simulink model "Model_accum"  (R2024a)
settings: Solver=FixedStepAuto  StartTime=0.0  StopTime=2000  RelTol=1e-3
undefined symbols (not defined in the file or in its folder): air_density, air_din_visc, air_pr, air_pr50, air_rashod, air_transmit, d, D, i_ph, L, lambda_alum, rho, Rzagr, TAM_spec_heat, thickness, vel_crist
settings Model: Creator=User  LastModifiedBy=User

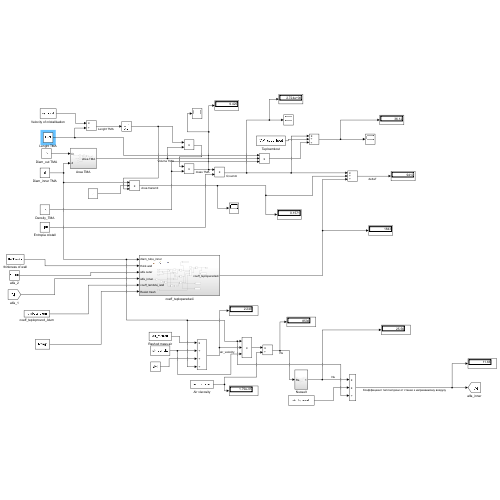
[thumbnail: Simulink's stored preview of the top-level diagram]
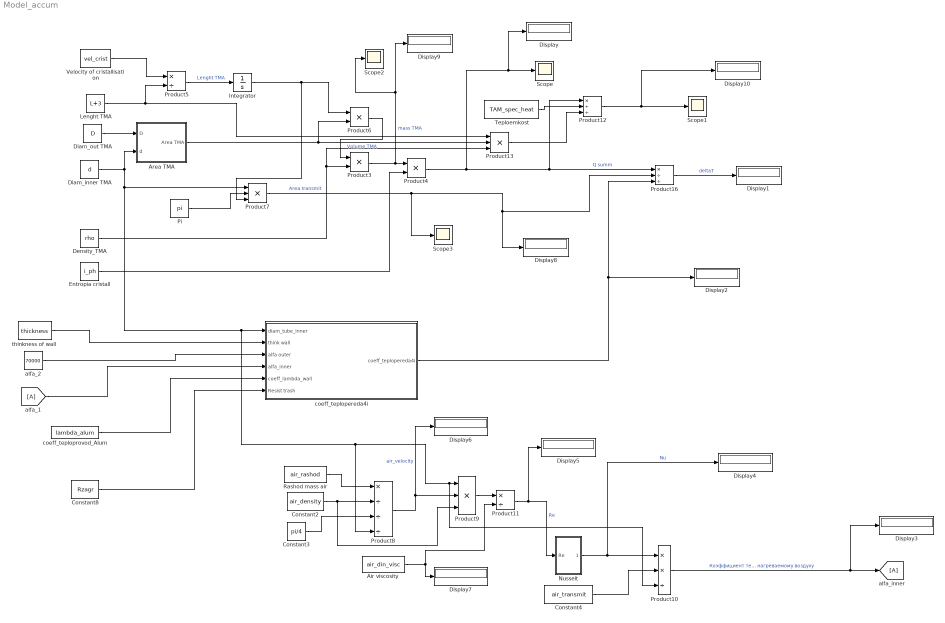
== system Model_accum ==
  Air viscosity : Constant  Value=air_din_visc
  Area TMA : Subsystem
  Constant2 : Constant  Value=air_density
  Constant3 : Constant  Value=pi/4
  Constant4 : Constant  Value=air_transmit
  Constant8 : Constant  Value=Rzagr
  Density_TMA : Constant  Value=rho
  Diam_inner TMA : Constant  Value=d
  Diam_out TMA : Constant  Value=D
  Display{,1..10} (11 alike) : Display
  Entropia cristall : Constant  Value=i_ph
  Integrator : Integrator  InitialCondition=0.001  LimitOutput=on  UpperSaturationLimit=1
  Lenght TMA : Constant  Value=L+3
  Nusselt : Subsystem
  Pi : Constant  Value=pi  OutDataTypeStr=Inherit: Inherit via back propagation
  Product10 : Product  Inputs=**/
  Product11 : Product  Inputs=*/
  Product12 : Product  Inputs=*//
  Product13 : Product  Inputs=3
  Product16 : Product  Inputs=*//
  Product3 : Product
  Product4 : Product
  Product5 : Product  Inputs=*/
  Product6 : Product
  Product7 : Product  Inputs=3
  Product8 : Product  Inputs=*///
  Product9 : Product  Inputs=3
  Rashod mass air : Constant  Value=air_rashod
  Scope{,1..3} (4 alike) : Scope
  Teploemkost : Constant  Value=TAM_spec_heat
  Velocity of cristallisation : Constant  Value=vel_crist
  alfa_1 : From
  alfa_2 : Constant  Value=70000
  alfa_inner : Goto
  coeff_teplopereda4i : Subsystem
  coeff_teploprovod_Alum : Constant  Value=lambda_alum
  thinkness of wall : Constant  Value=thickness
  wires:
  Lenght TMA/1 -> Product13/1, Product5/2
  Area TMA/1(Area TMA) -> Product6/2, Product13/2  "Volume TMA"
  Density_TMA/1 -> Product13/3, Product3/2
  Product3/1 -> Scope2/1, Display9/1, Product4/1  "mass TMA"
  Entropia cristall/1 -> Product4/2
  Product4/1 -> Product12/1, Product16/1, Scope/1, Display/1  "Q summ"
  Velocity of cristallisation/1 -> Product5/1
  Product5/1 -> Integrator/1  "Lenght TMA"
  Integrator/1 -> Product7/3, Product6/1
  Product6/1 -> Product3/1
  Product7/1 -> Scope3/1, Display8/1, Product16/2  "Area transmit"
  Product16/1 -> Display1/1  "deltaT"
  coeff_teplopereda4i/1(coeff_teplopereda4i) -> Product16/3, Display2/1
  thinkness of wall/1 -> coeff_teplopereda4i/2(think wall)
  alfa_2/1 -> coeff_teplopereda4i/3(alfa outer)
  alfa_1/1 -> coeff_teplopereda4i/4(alfa_inner)
  coeff_teploprovod_Alum/1 -> coeff_teplopereda4i/5(coeff_lambda_wall)
  Constant8/1 -> coeff_teplopereda4i/6(Resist trash)
  Diam_inner TMA/1 -> Product10/3, Product9/1, Product8/4, coeff_teplopereda4i/1(diam_tube_inner), Product7/1, Area TMA/2(d)
  Rashod mass air/1 -> Product8/1
  Constant2/1 -> Product9/3, Product8/2
  Constant3/1 -> Product8/3
  Product8/1 -> Display6/1, Product9/2  "air_velocity"
  Air viscosity/1 -> Product11/2, Display7/1
  Product11/1 -> Nusselt/1(Re), Display5/1  "Re"
  Nusselt/1(Out1) -> Display4/1, Product10/1  "Nu"
  Constant4/1 -> Product10/2
  Product10/1 -> alfa_inner/1, Display3/1  "Коэффициент теплоотдачи от стенки к нагреваемому воздуху"
  Product9/1 -> Product11/1
  Pi/1 -> Product7/2
  Teploemkost/1 -> Product12/2
  Product13/1 -> Product12/3
  Product12/1 -> Display10/1, Scope1/1
  Diam_out TMA/1 -> Area TMA/1(D)

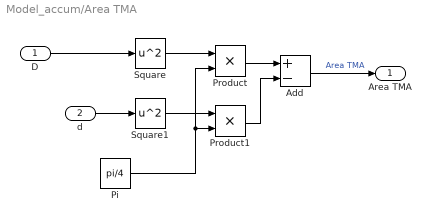
== system Model_accum/Area TMA ==
  D : Inport
  d : Inport  Port=2
  Add : Sum  Inputs=+-
  Pi : Constant  Value=pi/4  OutDataTypeStr=Inherit: Inherit via back propagation
  Product : Product
  Product1 : Product
  Square : Math  Operator=square
  Square1 : Math  Operator=square
  Area TMA : Outport
  wires:
  Square1/1 -> Product1/1
  Pi/1 -> Product/2, Product1/2
  Product1/1 -> Add/2
  D/1 -> Square/1
  Square/1 -> Product/1
  Add/1 -> Area TMA/1  "Area TMA"
  Product/1 -> Add/1
  d/1 -> Square1/1

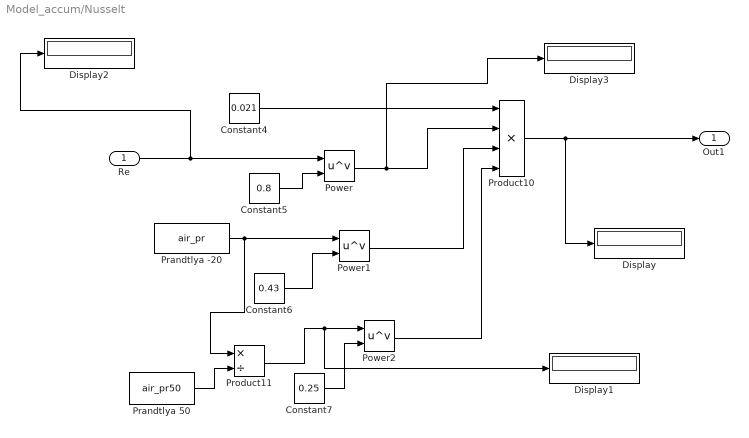
== system Model_accum/Nusselt ==
  Re : Inport
  Constant4 : Constant  Value=0.021
  Constant5 : Constant  Value=0.8
  Constant6 : Constant  Value=0.43
  Constant7 : Constant  Value=0.25
  Display{,1..3} (4 alike) : Display
  Power : Math  Operator=pow
  Power1 : Math  Operator=pow
  Power2 : Math  Operator=pow
  Prandtlya -20 : Constant  Value=air_pr
  Prandtlya 50 : Constant  Value=air_pr50
  Product10 : Product  Inputs=4
  Product11 : Product  Inputs=*/
  Out1 : Outport
  wires:
  Prandtlya -20/1 -> Product11/1, Power1/1
  Constant4/1 -> Product10/1
  Prandtlya 50/1 -> Product11/2
  Power1/1 -> Product10/3
  Constant5/1 -> Power/2
  Product11/1 -> Display1/1, Power2/1
  Power/1 -> Display3/1, Product10/2
  Constant6/1 -> Power1/2
  Constant7/1 -> Power2/2
  Power2/1 -> Product10/4
  Product10/1 -> Display/1, Out1/1
  Re/1 -> Display2/1, Power/1

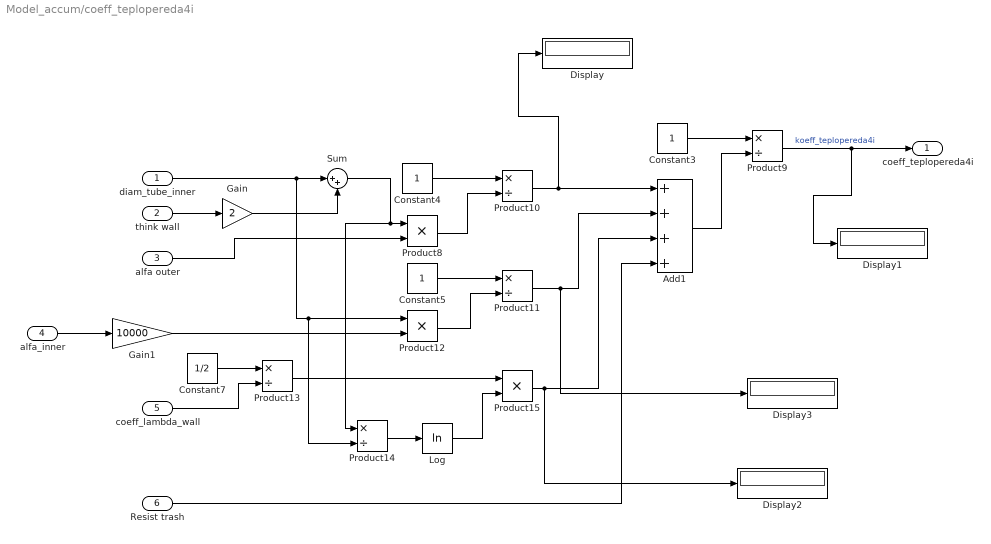
== system Model_accum/coeff_teplopereda4i ==
  diam_tube_inner : Inport
  think wall : Inport  Port=2
  alfa outer : Inport  Port=3
  alfa_inner : Inport  Port=4
  coeff_lambda_wall : Inport  Port=5
  Resist trash : Inport  Port=6
  Add1 : Sum  Inputs=++++
  Constant3 : Constant
  Constant4 : Constant
  Constant5 : Constant
  Constant7 : Constant  Value=1/2
  Display{,1..3} (4 alike) : Display
  Gain : Gain  Gain=2
  Gain1 : Gain  Gain=10000
  Log : Math  Operator=log
  Product{9..11,13..14} (5 alike) : Product  Inputs=*/
  Product12 : Product
  Product15 : Product
  Product8 : Product
  Sum : Sum  Inputs=|++
  coeff_teplopereda4i : Outport
  wires:
  diam_tube_inner/1 -> Product14/2, Product12/1, Sum/1
  Constant3/1 -> Product9/1
  think wall/1 -> Gain/1
  alfa_inner/1 -> Gain1/1
  Log/1 -> Product15/2
  Product13/1 -> Product15/1
  Product11/1 -> Display3/1, Add1/2
  Sum/1 -> Product14/1, Product8/1
  Resist trash/1 -> Add1/4
  Constant4/1 -> Product10/1
  Product12/1 -> Product11/2
  coeff_lambda_wall/1 -> Product13/2
  Product8/1 -> Product10/2
  Constant7/1 -> Product13/1
  Constant5/1 -> Product11/1
  Add1/1 -> Product9/2
  Product15/1 -> Display2/1, Add1/3
  Product14/1 -> Log/1
  Product10/1 -> Display/1, Add1/1
  alfa outer/1 -> Product8/2
  Product9/1 -> Display1/1, coeff_teplopereda4i/1  "koeff_teplopereda4i"
  Gain/1 -> Sum/2
  Gain1/1 -> Product12/2
